simulink model "PV_mppt_boost"  (R2018a)
settings: Solver=ode3  StartTime=0.0  StopTime=3.3  FixedStep=1e-4  RelTol=1e-3  EnableMultiTasking=on
undefined symbols (not defined in the file): a, C, Eg0, Gn, Isc, K, ki, L, n, Ns, q, R, Rs, Rsh, Tn, Voc
settings Model: Creator=PC  LastModifiedBy=yassine
settings OptimizationCC: LifeSpan=inf
settings DebuggingCC: SFUnexpectedBacktrackingDiag=warning  SFNoUnconditionalDefaultTransitionDiag=warning
settings CodeAppCC: StateflowObjectComments=on
settings GRTTargetCC: TargetLangStandard=C89/C90 (ANSI)
settings ConfigComp: CovMetricSettings=dw  CovSaveCumulativeToWorkspaceVar=on  CovSaveSingleToWorkspaceVar=on  CovExternalEMLEnable=off

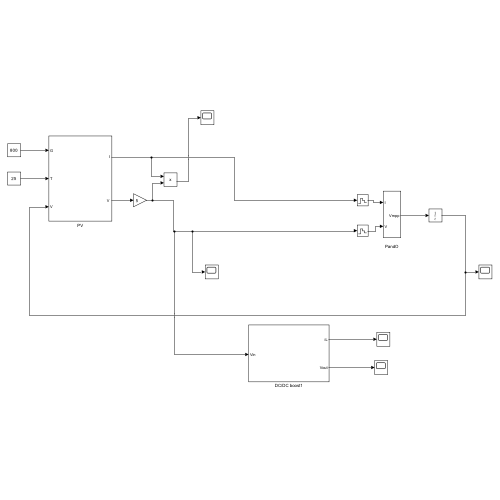
[thumbnail: Simulink's stored preview of the top-level diagram]
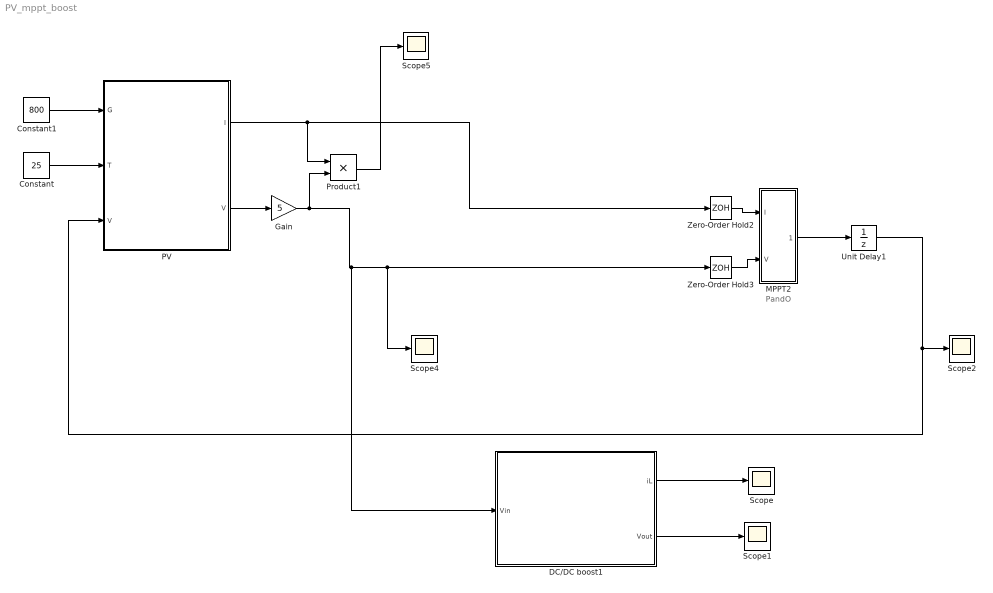
== system PV_mppt_boost ==
  note: PandO
  Constant : Constant  Value=25
  Constant1 : Constant  Value=800
  DC/DC boost1 : Subsystem  InitFcn=|
      | dv=0.5;
      | di=0.1;
      | F=20e3;
      | T=1/F;
      | Vs=230;
      | Vab=sqrt(3)*Vs;
      | Vdc=2*sqrt(2)*Vab/sqrt(3);
      | Vpv=131.5;
      | a=1-Vpv/Vdc;
      | Pn=200*5;
      | R=Vdc*Vdc/Pn;
      | L=0.5*Vpv*a*T/di;
      | C=0.5*Vdc*a*T/(dv*R);
  Gain : Gain  Gain=5
  MPPT2 : Subsystem
  PV : Subsystem  InitFcn=|
      | ki=.0032;
      | q=1.6e-19;
      | K=1.38e-23;
      | n=1.3;
      | Eg0=1.12;
      | Rs=.221;
      | Rsh=415.405;
      | Tn=298.15;
      | Gn=1000
      | Voc=32.9;
      | Isc=8.21;
      | Ns=54;
  Product1 : Product
  Scope{,1..2,4..5} (5 alike) : Scope
  Unit Delay1 : UnitDelay  SampleTime=1e-4  HasFrameUpgradeWarning=on
  Zero-Order Hold2 : ZeroOrderHold  SampleTime=1e-4
  Zero-Order Hold3 : ZeroOrderHold  SampleTime=1e-4
  wires:
  PV/2("V ") -> Gain/1
  MPPT2/1(Vmpp) -> Unit Delay1/1
  Zero-Order Hold2/1 -> MPPT2/1(I)
  Zero-Order Hold3/1 -> MPPT2/2(V)
  PV/1(I) -> Product1/1, Zero-Order Hold2/1
  Unit Delay1/1 -> Scope2/1, PV/3(V)
  Product1/1 -> Scope5/1
  Constant/1 -> PV/2(T)
  Constant1/1 -> PV/1(G)
  DC/DC boost1/1(iL) -> Scope/1
  DC/DC boost1/2(Vout) -> Scope1/1
  Gain/1 -> Product1/2, DC/DC boost1/1(Vin), Scope4/1, Zero-Order Hold3/1

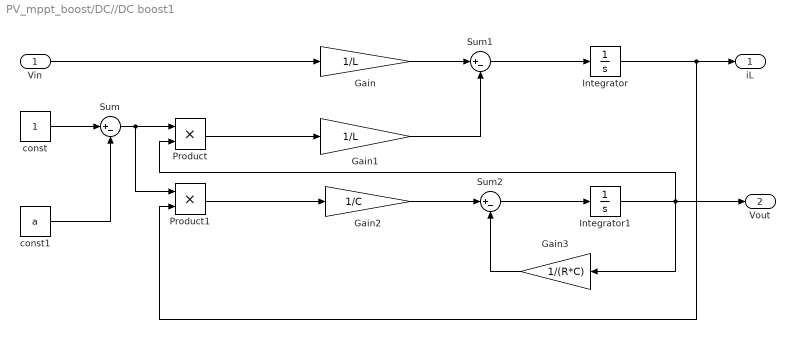
== system PV_mppt_boost/DC//DC boost1 ==
  Vin : Inport
  Gain : Gain  Gain=1/L
  Gain1 : Gain  Gain=1/L
  Gain2 : Gain  Gain=1/C
  Gain3 : Gain  Gain=1/(R*C)
  Integrator : Integrator
  Integrator1 : Integrator
  Product : Product
  Product1 : Product
  Sum : Sum  Inputs=|+-
  Sum1 : Sum  Inputs=|+-
  Sum2 : Sum  Inputs=|+-
  const : Constant
  const1 : Constant  Value=a
  iL : Outport
  Vout : Outport  Port=2
  wires:
  Gain3/1 -> Sum2/2
  Integrator1/1 -> Vout/1, Product/2, Gain3/1
  Sum2/1 -> Integrator1/1
  Integrator/1 -> iL/1, Product1/2
  Vin/1 -> Gain/1
  const/1 -> Sum/1
  Product1/1 -> Gain2/1
  Product/1 -> Gain1/1
  Sum1/1 -> Integrator/1
  Gain1/1 -> Sum1/2
  Sum/1 -> Product/1, Product1/1
  Gain2/1 -> Sum2/1
  Gain/1 -> Sum1/1
  const1/1 -> Sum/2

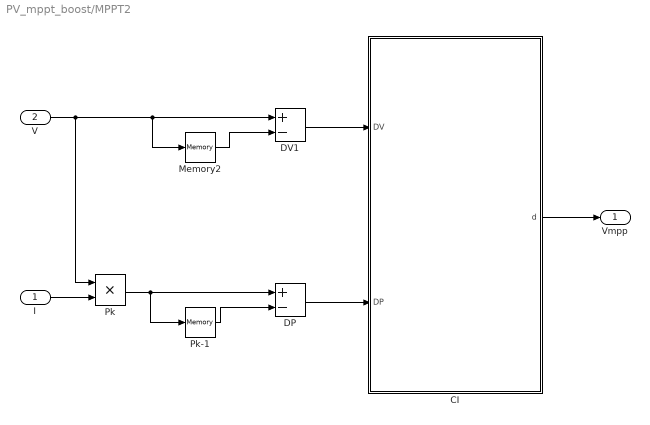
== system PV_mppt_boost/MPPT2 ==
  I : Inport
  V : Inport  Port=2
  CI : MATLAB Function  TreatAsAtomicUnit=on
  DP : Sum  Inputs=+-
  DV1 : Sum  Inputs=+-
  Memory2 : Memory
  Pk : Product  Inputs=**
  Pk-1 : Memory  InitialCondition=-0.1
  Vmpp : Outport
  wires:
  DP/1 -> CI/2(DP)
  DV1/1 -> CI/1(DV)
  CI/1(d) -> Vmpp/1
  Pk-1/1 -> DP/2
  Pk/1 -> Pk-1/1, DP/1
  V/1 -> Pk/1, Memory2/1, DV1/1
  Memory2/1 -> DV1/2
  I/1 -> Pk/2

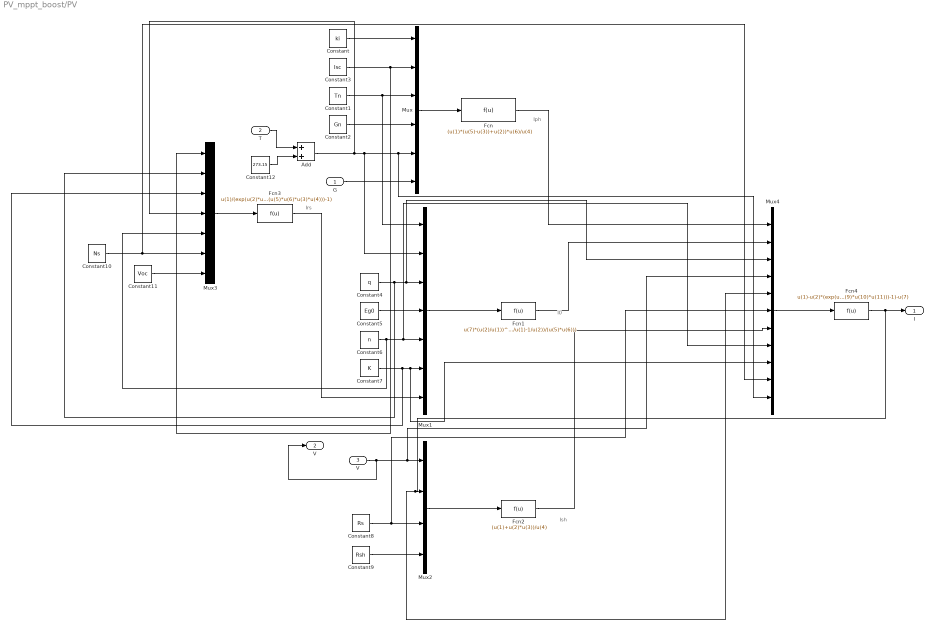
== system PV_mppt_boost/PV ==
  note: Irs
  note: Ish
  note: Iph
  note: I0
  G : Inport
  T : Inport  Port=2
  V : Inport  Port=3
  Add : Sum
  Constant : Constant  Value=ki
  Constant1 : Constant  Value=Tn
  Constant10 : Constant  Value=Ns
  Constant11 : Constant  Value=Voc
  Constant12 : Constant  Value=273.15
  Constant2 : Constant  Value=Gn
  Constant3 : Constant  Value=Isc
  Constant4 : Constant  Value=q
  Constant5 : Constant  Value=Eg0
  Constant6 : Constant  Value=n
  Constant7 : Constant  Value=K
  Constant8 : Constant  Value=Rs
  Constant9 : Constant  Value=Rsh
  Fcn : Fcn  Expr=(u(1)*(u(5)-u(3))+u(2))*u(6)/u(4)
  Fcn1 : Fcn  Expr=u(7)*(u(2)/u(1))^3*exp(u(3)*u(4)*(1/u(1)-1/u(2))/(u(5)*u(6)))
  Fcn2 : Fcn  Expr=(u(1)+u(2)*u(3))/u(4)
  Fcn3 : Fcn  Expr=u(1)/(exp(u(2)*u(7)/(u(5)*u(6)*u(3)*u(4)))-1)
  Fcn4 : Fcn  Expr=u(1)-u(2)*(exp(u(3)*(u(4)+u(5)*u(6))/(u(8)*u(9)*u(10)*u(11)))-1)-u(7)
  Mux : Mux  Inputs=6
  Mux1 : Mux  Inputs=7
  Mux2 : Mux
  Mux3 : Mux  Inputs=7
  Mux4 : Mux  Inputs=11
  I : Outport
  "V " : Outport  Port=2
  wires:
  Constant11/1 -> Mux3/7
  Fcn4/1 -> I/1, Mux4/5, Mux2/2
  Mux1/1 -> Fcn1/1
  Constant9/1 -> Mux2/4
  Constant7/1 -> Mux4/9, Mux1/6, Mux3/3
  Add/1 -> Mux4/11, Mux/5, Mux1/2, Mux3/4
  Mux2/1 -> Fcn2/1
  Fcn2/1 -> Mux4/7
  Constant4/1 -> Mux4/3, Mux1/3, Mux3/2
  Fcn1/1 -> Mux4/2
  Constant/1 -> Mux/1
  Fcn3/1 -> Mux1/7
  G/1 -> Mux/6
  Constant5/1 -> Mux1/4
  Constant1/1 -> Mux1/1, Mux/3
  Constant6/1 -> Mux4/8, Mux1/5, Mux3/5
  Constant10/1 -> Mux4/10, Mux3/6
  Constant3/1 -> Mux/2, Mux3/1
  Mux3/1 -> Fcn3/1
  Fcn/1 -> Mux4/1
  Constant8/1 -> Mux4/6, Mux2/3
  Mux/1 -> Fcn/1
  Constant2/1 -> Mux/4
  V/1 -> "V "/1, Mux4/4, Mux2/1
  Mux4/1 -> Fcn4/1
  Constant12/1 -> Add/2
  T/1 -> Add/1

== matlab function PV_mppt_boost/MPPT2/CI ==
  data: DV input; DP input; d output
function d=PO(DV,DP)
persistent   m ;

if isempty(m)
    m=26.3;
end

if(DP==0)
else
    if(DP>0)
        if(DV>0)
                m=m+0.00001;
            else
                m=m-0.00001;
           end 
       else
        if(DV>0)
                m=m-0.00001;
            else
                m=m+0.00001;
        end
    end
end
if(m<25)
    m=25;
end
if(m>33)
    m=33;
end

d=m;
end
